simulink model "NeuralNetUnitLDC"  (R2018a)
settings: Solver=VariableStepAuto  StartTime=0.0  StopTime=20  RelTol=1e-3
values from neighbouring files (symbols this model uses):
  B = 0.5    [Parameters.m]    (also in Untitled2.m = 68530.7; Untitled3.m = 68530.7)
  b = 0.05    [Parameters.m]
  l = 0.6    [Parameters.m]
  m = 0.250    (= 0.25)    [Parameters.m]
  R = 0.1    [Parameters.m]
settings Model: Creator=Therecia  LastModifiedBy=nyandoro
settings CodeAppCC: StateflowObjectComments=on

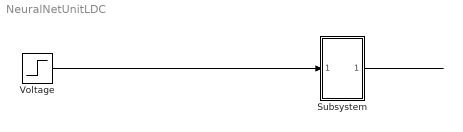
== system NeuralNetUnitLDC ==
  Subsystem : Subsystem
      mask DialogControl Control2 Prompt: BlackBox
  Voltage : Step  SampleTime=0
  wires:
  Voltage/1 -> Subsystem/1(In1)
  Subsystem/1(Out1) -> ?

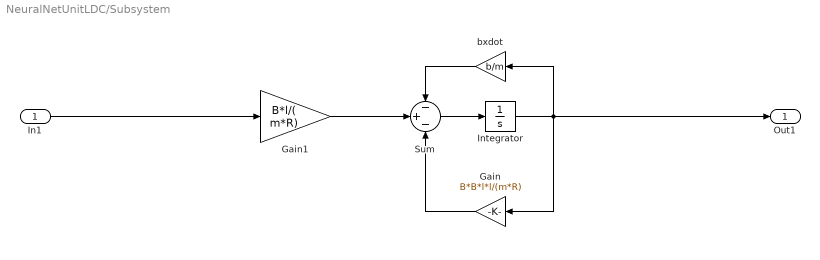
== system NeuralNetUnitLDC/Subsystem ==
  In1 : Inport
  Gain : Gain  Gain=B*B*l*l/(m*R)
  Gain1 : Gain  Gain=B*l/( m*R)
  Integrator : Integrator
  Sum : Sum  Inputs=-+-
  bxdot : Gain  Gain=b/m
  Out1 : Outport
  wires:
  In1/1 -> Gain1/1
  Sum/1 -> Integrator/1
  Gain/1 -> Sum/3
  Integrator/1 -> Out1/1, bxdot/1, Gain/1
  Gain1/1 -> Sum/2
  bxdot/1 -> Sum/1
